simulink model "mvdr_4x4_partial_systolic"  (R2023a)
settings: Solver=FixedStepDiscrete  StartTime=0.0  StopTime=stoptime  RelTol=1e-3
InitFcn:
  | model_init
values from neighbouring files (symbols this model uses):
  diagLoading = 5e-3    (= 0.005)    [model_init.m]
  movavg_bitshift = nextpow2(windowSize)    [model_init.m]
  mvdrPipelineDelay = covMatDelay+movAvgDelay+matrixSolveDelay+normResponseDelay    [model_init.m]
  numArrayElements = 4    [model_init.m]
  reciprocalDelay = nextpow2(reciprocalin_dt.WordLength) + 1 + reciprocalin_dt.WordLength + 2      - strcmp(reciprocalin_dt.Signedness,'Signed') + 7    [model_init.m]
  sv = double(fi(signalWeights, sv_dt))    [model_init.m]
  sv_dt = fixdt(1,18,16)    [model_init.m]
  windowSize = 4096    [model_init.m]
undefined symbols (not defined in the file or in its folder): NumBits1, NumBits2
libraries: hdlsllib x17, simulink x6, dspsrcs4 x2, embsystolicmatrixops x1, embreciprocals x1
Description:
  | MVDR HDL 4x4 systolic testbench
settings Model: DataTypeOverride=Off  Creator=The MathWorks, Inc.  LastModifiedBy=tmealey
settings SolverCC: AlgebraicLoopSolver=TrustRegion
settings DataIOCC: LimitDataPoints=on  SaveFormat=Array  SaveOutput=off  SignalLogging=off  SaveTime=off
settings OptimizationCC: BlockReduction=off  ConditionallyExecuteInputs=off  DefaultParameterBehavior=Inlined  InheritOutputTypeSmallerThanSingle=on  LifeSpan=inf
settings DebuggingCC: ReadBeforeWriteMsg=DisableAll  WriteAfterWriteMsg=DisableAll  WriteAfterReadMsg=DisableAll  AlgebraicLoopMsg=error  UnderspecifiedInitializationDetection=Classic  MergeDetectMultiDrivingBlocksExec=none  SolverPrmCheckMsg=warning  SingleTaskRateTransMsg=error  ParameterPrecisionLossMsg=none  UnconnectedInputMsg=warning  UnconnectedOutputMsg=warning  UnconnectedLineMsg=warning  AllowSymbolicDim=off  SFUnexpectedBacktrackingDiag=warning  SFNoUnconditionalDefaultTransitionDiag=warning  SFExecutionAtInitializationDiag=none  ArithmeticOperatorsInVariantConditions=warning
settings HardwareCC: ProdBitPerPointer=32  ProdBitPerSizeT=32  ProdBitPerPtrDiffT=32  ProdLargestAtomicFloat=None  ProdIntDivRoundTo=Undefined  ProdEndianess=Unspecified  ProdWordSize=32  ProdHWDeviceType=ASIC/FPGA->ASIC/FPGA  TargetBitPerPointer=64  TargetBitPerSizeT=64  TargetBitPerPtrDiffT=64  TargetLongLongMode=on  TargetIntDivRoundTo=Zero  TargetEndianess=LittleEndian  TargetWordSize=64  TargetHWDeviceType=Custom Processor->MATLAB Host Computer  ProdEqTarget=off
settings ModelReferenceCC: EnableRefExpFcnMdlSchedulingChecks=on  PropagateSignalLabelsOutOfModel=off
settings SFSimCC: SimUseLocalCustomCode=off  CustomCodeUndefinedFunction=UseInterfaceOnly
settings RTWCC: RTWUseLocalCustomCode=off  DLArmComputeVersion=19.05
settings CodeAppCC: StateflowObjectComments=on
settings GRTTargetCC: TargetLangStandard=C89/C90 (ANSI)
settings ConfigComp: CovMetricSettings=dw  CovSaveCumulativeToWorkspaceVar=on  CovSaveSingleToWorkspaceVar=on  CovExternalEMLEnable=off  CovSFcnEnable=off

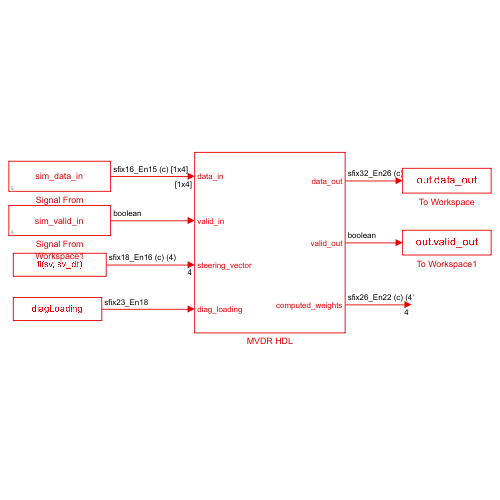
[thumbnail: Simulink's stored preview of the top-level diagram]
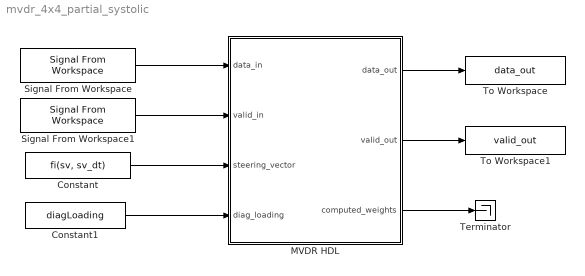
== system mvdr_4x4_partial_systolic ==
  Constant : Constant  Value=fi(sv, sv_dt)  SampleTime=1
  Constant1 : Constant  Value=diagLoading  OutDataTypeStr=matrixdivin_dt  SampleTime=-1
  MVDR HDL : Subsystem
  Signal From Workspace : dspsrcs4/Signal From Workspace  X=sim_data_in  Ts=1  nsamps=1  OutputAfterFinalValue=Setting to zero  ignoreOrWarnInputAndFrameLengths=off  OutputFrames=off
  Signal From Workspace1 : dspsrcs4/Signal From Workspace  X=sim_valid_in  Ts=1  nsamps=1  OutputAfterFinalValue=Setting to zero  ignoreOrWarnInputAndFrameLengths=off  OutputFrames=off
  Terminator : Terminator
  To Workspace : ToWorkspace  VariableName=data_out  SampleTime=-1
      settings: Save2DSignal=2-D array (concatenate along first dimension)
  To Workspace1 : ToWorkspace  VariableName=valid_out  SampleTime=-1
      settings: Save2DSignal=2-D array (concatenate along first dimension)
  wires:
  MVDR HDL/2(valid_out) -> To Workspace1/1
  MVDR HDL/1(data_out) -> To Workspace/1
  Constant/1 -> MVDR HDL/3(steering_vector)
  Signal From Workspace/1 -> MVDR HDL/1(data_in)
  Signal From Workspace1/1 -> MVDR HDL/2(valid_in)
  MVDR HDL/3(computed_weights) -> Terminator/1
  Constant1/1 -> MVDR HDL/4(diag_loading)

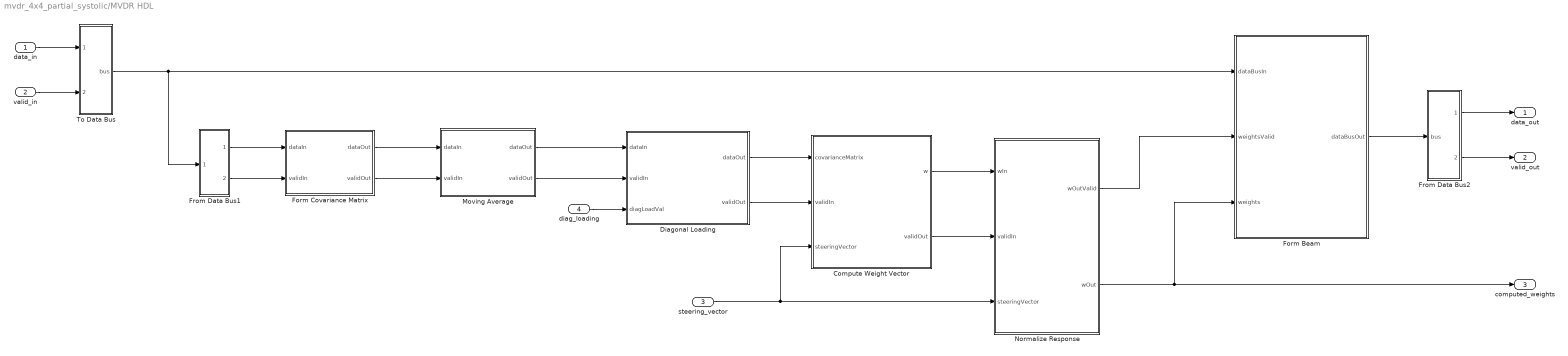
== system mvdr_4x4_partial_systolic/MVDR HDL ==
  data_in : Inport
  valid_in : Inport  Port=2
  steering_vector : Inport  Port=3
  diag_loading : Inport  Port=4
  Compute Weight Vector : Subsystem
  Diagonal Loading : Subsystem
  Form Beam : Subsystem
  Form Covariance Matrix : Subsystem
  From Data Bus1 : Subsystem
  From Data Bus2 : Subsystem
  Moving Average : Subsystem
  Normalize Response : Subsystem
  To Data Bus : Subsystem
  data_out : Outport
  valid_out : Outport  Port=2
  computed_weights : Outport  Port=3
  wires:
  valid_in/1 -> To Data Bus/2(valid)
  Form Covariance Matrix/2(validOut) -> Moving Average/2(validIn)
  Compute Weight Vector/1(w) -> Normalize Response/1(wIn)
  steering_vector/1 -> Normalize Response/3(steeringVector), Compute Weight Vector/3(steeringVector)
  data_in/1 -> To Data Bus/1(data)
  Form Covariance Matrix/1(dataOut) -> Moving Average/1(dataIn)
  To Data Bus/1(bus) -> From Data Bus1/1(bus), Form Beam/1(dataBusIn)
  Compute Weight Vector/2(validOut) -> Normalize Response/2(validIn)
  From Data Bus1/1(data) -> Form Covariance Matrix/1(dataIn)
  From Data Bus1/2(valid) -> Form Covariance Matrix/2(validIn)
  Form Beam/1(dataBusOut) -> From Data Bus2/1(bus)
  From Data Bus2/1(data) -> data_out/1
  From Data Bus2/2(valid) -> valid_out/1
  Diagonal Loading/2(validOut) -> Compute Weight Vector/2(validIn)
  Moving Average/2(validOut) -> Diagonal Loading/2(validIn)
  Moving Average/1(dataOut) -> Diagonal Loading/1(dataIn)
  Diagonal Loading/1(dataOut) -> Compute Weight Vector/1(covarianceMatrix)
  Normalize Response/2(wOut) -> computed_weights/1, Form Beam/3(weights)
  Normalize Response/1(wOutValid) -> Form Beam/2(weightsValid)
  diag_loading/1 -> Diagonal Loading/3(diagLoadVal)

== system mvdr_4x4_partial_systolic/MVDR HDL/Compute Weight Vector ==
  covarianceMatrix : Inport
  validIn : Inport  Port=2
  steeringVector : Inport  Port=3
  Complex Partial-Systolic Matrix Solve Using QR Decomposition : embsystolicmatrixops/Complex Partial-Systolic Matrix Solve Using QR Decomposition  m=4  n=4  p=1  regularizationParameter=0  OutputType=matrixdivbacksub_dt
  Constant : Constant  Value=false  SampleTime=-1
  Data Type Conversion2 : DataTypeConversion  OutDataTypeStr=matrixdivin_dt  SaturateOnIntegerOverflow=off  RndMeth=Floor
  Deserialize Output Data : Subsystem
  Reshape1 : Reshape  OutputDimensionality=Column vector (2-D)  OutputDimensions=[4,4]
  Serialize Input Data : Subsystem
  w : Outport
  validOut : Outport  Port=2
  wires:
  steeringVector/1 -> Data Type Conversion2/1
  Data Type Conversion2/1 -> Reshape1/1
  validIn/1 -> Serialize Input Data/3(validIn)
  Constant/1 -> Complex Partial-Systolic Matrix Solve Using QR Decomposition/4
  Serialize Input Data/3(validOut) -> Complex Partial-Systolic Matrix Solve Using QR Decomposition/3  "matrixSolveValidIn"
  Complex Partial-Systolic Matrix Solve Using QR Decomposition/3 -> Serialize Input Data/4(readyIn)  "matrixSolveReady"
  Serialize Input Data/1(AOut) -> Complex Partial-Systolic Matrix Solve Using QR Decomposition/1
  Reshape1/1 -> Serialize Input Data/2(BIn)
  Complex Partial-Systolic Matrix Solve Using QR Decomposition/1 -> Deserialize Output Data/1(dataIn)
  Complex Partial-Systolic Matrix Solve Using QR Decomposition/2 -> Deserialize Output Data/2(validIn)  "matrixSolveValidOut"
  Deserialize Output Data/1(dataOut) -> w/1
  Deserialize Output Data/2(validOut) -> validOut/1
  Serialize Input Data/2(BOut) -> Complex Partial-Systolic Matrix Solve Using QR Decomposition/2
  covarianceMatrix/1 -> Serialize Input Data/1(AIn)

== system mvdr_4x4_partial_systolic/MVDR HDL/Diagonal Loading ==
  dataIn : Inport
  validIn : Inport  Port=2
  diagLoadVal : Inport  Port=3
  Add : Sum
  Data Type Conversion1 : DataTypeConversion  OutDataTypeStr=matrixdivin_dt  SaturateOnIntegerOverflow=off  RndMeth=Floor
  Delay3 : Delay  DelayLength=1
  Delay6 : Delay  DelayLength=1
  Generate Loading Eye Matrix : MATLAB Function  TreatAsAtomicUnit=on
  Reshape1 : Reshape  OutputDimensions=[4,4]
  To Workspace2 : ToWorkspace  VariableName=Ecx_loaded  SampleTime=-1
      settings: Save2DSignal=2-D array (concatenate along first dimension)
  dataOut : Outport
  validOut : Outport  Port=2
  wires:
  Reshape1/1 -> To Workspace2/1
  Data Type Conversion1/1 -> dataOut/1, Reshape1/1
  Delay3/1 -> Data Type Conversion1/1
  dataIn/1 -> Add/2
  Generate Loading Eye Matrix/1(out) -> Add/1
  Add/1 -> Delay3/1
  Delay6/1 -> validOut/1
  diagLoadVal/1 -> Generate Loading Eye Matrix/1(in)
  validIn/1 -> Delay6/1

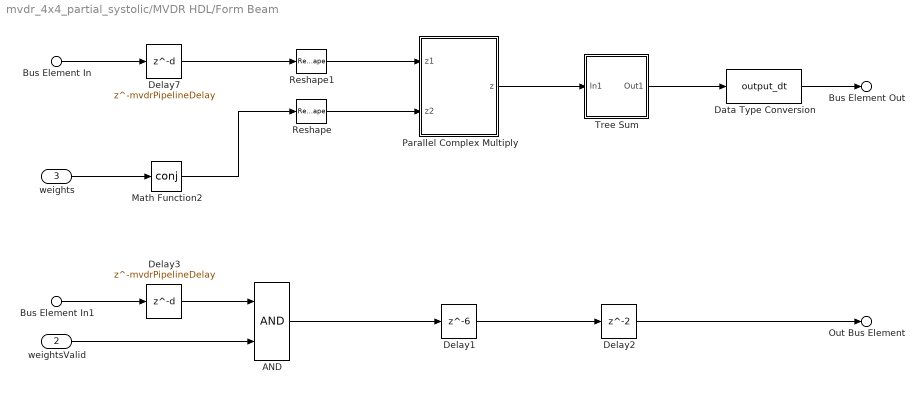
== system mvdr_4x4_partial_systolic/MVDR HDL/Form Beam ==
  Bus Element In : Inport  PortName=dataBusIn  Element=data
  Bus Element In1 : Inport  PortName=dataBusIn  Element=valid
  weightsValid : Inport  Port=2
  weights : Inport  Port=3
  AND : Logic  IconShape=distinctive  AllPortsSameDT=off  OutDataTypeStr=boolean
  Data Type Conversion : DataTypeConversion  OutDataTypeStr=output_dt  SaturateOnIntegerOverflow=off  RndMeth=Floor
  Delay1 : Delay  DelayLength=6
  Delay2 : Delay
  Delay3 : Delay  DelayLength=mvdrPipelineDelay
  Delay7 : Delay  DelayLength=mvdrPipelineDelay
  Math Function2 : Math  Operator=conj
  Parallel Complex Multiply : Subsystem  TreatAsAtomicUnit=on
  Reshape : Reshape
  Reshape1 : Reshape
  Tree Sum : Subsystem
  Bus Element Out : Outport  PortName=dataBusOut  Element=data
  Out Bus Element : Outport  PortName=dataBusOut  Element=valid
  wires:
  Parallel Complex Multiply/1(z) -> Tree Sum/1(In1)
  Tree Sum/1(Out1) -> Data Type Conversion/1
  Math Function2/1 -> Reshape/1
  weights/1 -> Math Function2/1
  Reshape/1 -> Parallel Complex Multiply/2(z2)
  Reshape1/1 -> Parallel Complex Multiply/1(z1)
  Data Type Conversion/1 -> Bus Element Out/1
  Delay2/1 -> Out Bus Element/1
  Delay1/1 -> Delay2/1
  Bus Element In1/1 -> Delay3/1
  Bus Element In/1 -> Delay7/1
  Delay7/1 -> Reshape1/1
  Delay3/1 -> AND/1
  weightsValid/1 -> AND/2
  AND/1 -> Delay1/1

== system mvdr_4x4_partial_systolic/MVDR HDL/Form Covariance Matrix ==
  dataIn : Inport
  validIn : Inport  Port=2
  Conj : Math  Operator=conj  SaturateOnIntegerOverflow=off
  Data Type Conversion : DataTypeConversion  OutDataTypeStr=covmat_dt  SaturateOnIntegerOverflow=off  RndMeth=Floor
  Data Type Conversion1 : DataTypeConversion  OutDataTypeStr=adc_dt  SaturateOnIntegerOverflow=off  RndMeth=Floor
  Delay : Delay  DelayLength=6
  Matrix Multiply Partitioned : Subsystem  TreatAsAtomicUnit=on
  Reshape : Reshape
  dataOut : Outport
  validOut : Outport  Port=2
  wires:
  validIn/1 -> Delay/1
  dataIn/1 -> Data Type Conversion1/1
  Reshape/1 -> Conj/1, Matrix Multiply Partitioned/1(x)  "x"
  Matrix Multiply Partitioned/1(C) -> Data Type Conversion/1  "x * x'"
  Delay/1 -> validOut/1
  Conj/1 -> Matrix Multiply Partitioned/2(x_conj)
  Data Type Conversion1/1 -> Reshape/1
  Data Type Conversion/1 -> dataOut/1

== system mvdr_4x4_partial_systolic/MVDR HDL/From Data Bus1 ==
  bus : Inport
  Bus Selector : BusSelector  OutputSignals=data,valid
  data : Outport
  valid : Outport  Port=2
  wires:
  bus/1 -> Bus Selector/1
  Bus Selector/1 -> data/1  "<data>"
  Bus Selector/2 -> valid/1  "<valid>"

== system mvdr_4x4_partial_systolic/MVDR HDL/From Data Bus2 ==
  bus : Inport
  Bus Selector : BusSelector  OutputSignals=data,valid
  data : Outport
  valid : Outport  Port=2
  wires:
  Bus Selector/2 -> valid/1  "<valid>"
  Bus Selector/1 -> data/1  "<data>"
  bus/1 -> Bus Selector/1

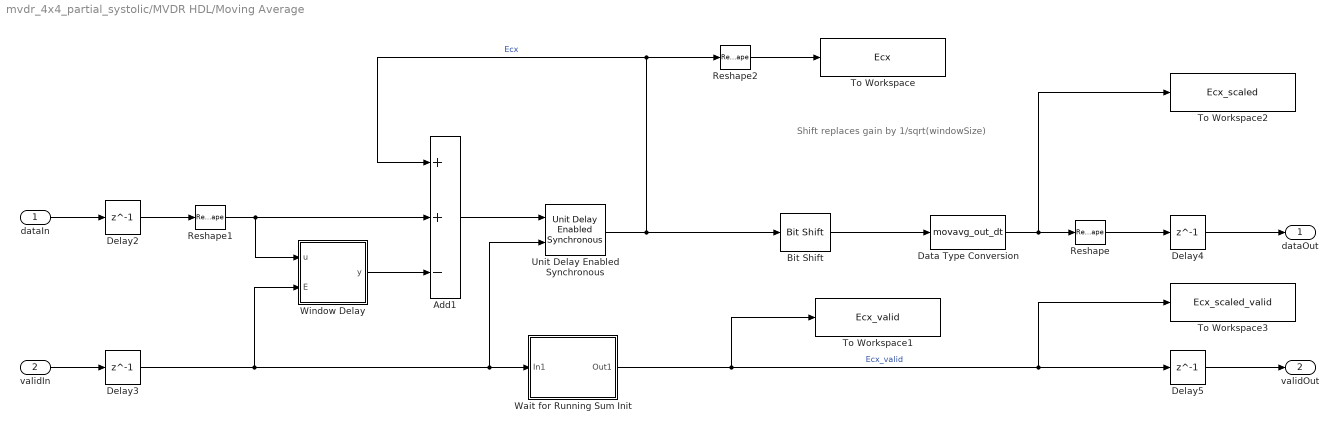
== system mvdr_4x4_partial_systolic/MVDR HDL/Moving Average ==
  note: Shift replaces gain by 1/sqrt(windowSize)
  dataIn : Inport
  validIn : Inport  Port=2
  Add1 : Sum  Inputs=++-  AccumDataTypeStr=movavg_accum_dt  OutDataTypeStr=Inherit: Same as accumulator
  Bit Shift : hdlsllib/Logic and Bit Operations/Bit Shift  mode=Shift Right Arithmetic  N=movavg_bitshift
  Data Type Conversion : DataTypeConversion  OutDataTypeStr=movavg_out_dt  SaturateOnIntegerOverflow=off  RndMeth=Floor
  Delay{2..5} (4 alike) : Delay  DelayLength=1
  Reshape : Reshape  OutputDimensionality=Customize  OutputDimensions=[4,4]
  Reshape1 : Reshape  OutputDimensions=[4,4]
  Reshape2 : Reshape  OutputDimensions=[4,4]
  To Workspace : ToWorkspace  VariableName=Ecx  SampleTime=-1
      settings: Save2DSignal=2-D array (concatenate along first dimension)
  To Workspace1 : ToWorkspace  VariableName=Ecx_valid  SampleTime=-1
      settings: Save2DSignal=2-D array (concatenate along first dimension)
  To Workspace2 : ToWorkspace  VariableName=Ecx_scaled  SampleTime=-1
      settings: Save2DSignal=2-D array (concatenate along first dimension)
  To Workspace3 : ToWorkspace  VariableName=Ecx_scaled_valid  SampleTime=-1
      settings: Save2DSignal=2-D array (concatenate along first dimension)
  Unit Delay Enabled Synchronous : hdlsllib/Discrete/Unit Delay Enabled Synchronous  InitialCondition=0.0  SampleTime=-1
  Wait for Running Sum Init : Subsystem
  Window Delay : Subsystem
  dataOut : Outport
  validOut : Outport  Port=2
  wires:
  Bit Shift/1 -> Data Type Conversion/1
  Unit Delay Enabled Synchronous/1 -> Bit Shift/1, Add1/1, Reshape2/1  "Ecx"
  Add1/1 -> Unit Delay Enabled Synchronous/1
  dataIn/1 -> Delay2/1
  validIn/1 -> Delay3/1
  Delay2/1 -> Reshape1/1
  Delay4/1 -> dataOut/1
  Delay5/1 -> validOut/1
  Delay3/1 -> Window Delay/2(E), Unit Delay Enabled Synchronous/2, Wait for Running Sum Init/1(In1)
  Wait for Running Sum Init/1(Out1) -> To Workspace1/1, To Workspace3/1, Delay5/1  "Ecx_valid"
  Data Type Conversion/1 -> To Workspace2/1, Reshape/1
  Reshape/1 -> Delay4/1
  Reshape1/1 -> Window Delay/1(u), Add1/2
  Window Delay/1(y) -> Add1/3
  Reshape2/1 -> To Workspace/1

== system mvdr_4x4_partial_systolic/MVDR HDL/Normalize Response ==
  note: This subsystem scales the weight vector to ensure unit gain in the target direction.
  wIn : Inport
  validIn : Inport  Port=2
  steeringVector : Inport  Port=3
  MVDR Weight Update : Subsystem
  Set Latch : Subsystem
  Unit Delay Enabled Synchronous : hdlsllib/Discrete/Unit Delay Enabled Synchronous  InitialCondition=0.0  SampleTime=-1
  wOutValid : Outport
  wOut : Outport  Port=2
  wires:
  steeringVector/1 -> MVDR Weight Update/1(sv)
  wIn/1 -> MVDR Weight Update/2(wp)
  MVDR Weight Update/1(w) -> Unit Delay Enabled Synchronous/1
  MVDR Weight Update/2(validOut) -> Set Latch/1(S), Unit Delay Enabled Synchronous/2
  Unit Delay Enabled Synchronous/1 -> wOut/1
  validIn/1 -> MVDR Weight Update/3(validIn)
  Set Latch/1(Q) -> wOutValid/1

== system mvdr_4x4_partial_systolic/MVDR HDL/To Data Bus ==
  data : Inport
  valid : Inport  Port=2
  Bus Creator : BusCreator  Inputs=2
  bus : Outport
  wires:
  data/1 -> Bus Creator/1  "data"
  Bus Creator/1 -> bus/1
  valid/1 -> Bus Creator/2  "valid"

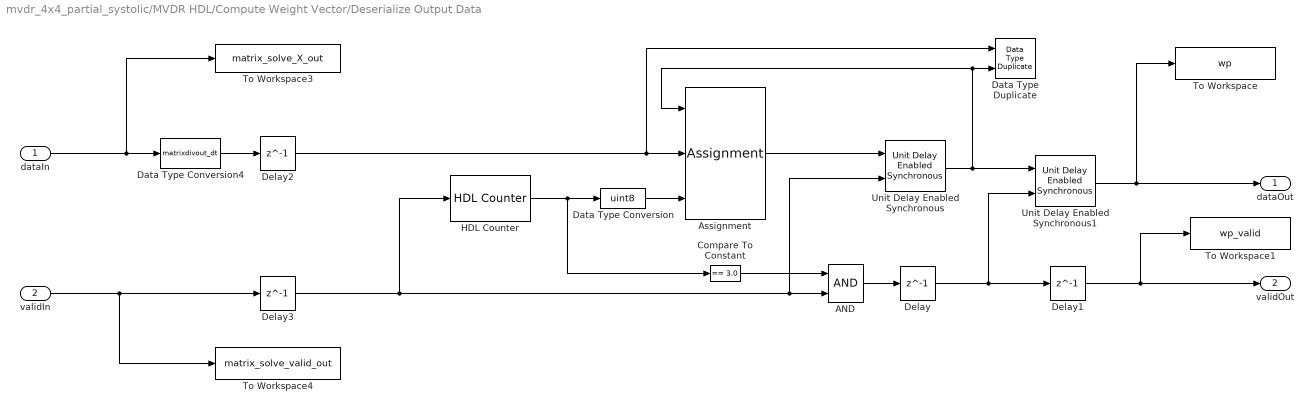
== system mvdr_4x4_partial_systolic/MVDR HDL/Compute Weight Vector/Deserialize Output Data ==
  dataIn : Inport
  validIn : Inport  Port=2
  AND : Logic  IconShape=distinctive  AllPortsSameDT=off  OutDataTypeStr=boolean
  Assignment : Assignment  IndexMode=Zero-based  DiagnosticForDimensions=Warning  IndexOptions=Index vector (port)  Indices=1  OutputSizes=4
  Compare To Constant : simulink/Logic and Bit Operations/Compare To Constant  relop===  const=3.0  OutDataTypeStr=boolean
  Data Type Duplicate : DataTypeDuplicate
  Data Type Conversion : DataTypeConversion  OutDataTypeStr=uint8  SaturateOnIntegerOverflow=off  RndMeth=Floor
  Data Type Conversion4 : DataTypeConversion  OutDataTypeStr=matrixdivout_dt  RndMeth=Convergent  SaturateOnIntegerOverflow=off
  Delay{,1..3} (4 alike) : Delay  DelayLength=1
  HDL Counter : hdlsllib/Sources/HDL Counter  CountType=Free running  CountInit=0  CountStep=1  CountMax=25  CountFromType=Initial value  CountFrom=0  CountResetPort=off  CountLoadPort=off  CountEnbPort=on  CountDirPort=off  CountHitOutputPort=off  CountDataType=Unsigned  CountWordLen=2  CountFracLen=0  CountSampTime=1
  To Workspace : ToWorkspace  VariableName=wp  SampleTime=-1
      settings: Save2DSignal=2-D array (concatenate along first dimension)
  To Workspace1 : ToWorkspace  VariableName=wp_valid  SampleTime=-1
      settings: Save2DSignal=2-D array (concatenate along first dimension)
  To Workspace3 : ToWorkspace  VariableName=matrix_solve_X_out  SampleTime=-1
      settings: Save2DSignal=2-D array (concatenate along first dimension)
  To Workspace4 : ToWorkspace  VariableName=matrix_solve_valid_out  SampleTime=-1
      settings: Save2DSignal=2-D array (concatenate along first dimension)
  Unit Delay Enabled Synchronous : hdlsllib/Discrete/Unit Delay Enabled Synchronous  InitialCondition=complex(zeros(4,1))  SampleTime=-1
  Unit Delay Enabled Synchronous1 : hdlsllib/Discrete/Unit Delay Enabled Synchronous  InitialCondition=0  SampleTime=-1
  dataOut : Outport
  validOut : Outport  Port=2
  wires:
  AND/1 -> Delay/1
  HDL Counter/1 -> Compare To Constant/1, Data Type Conversion/1
  dataIn/1 -> Data Type Conversion4/1, To Workspace3/1
  Compare To Constant/1 -> AND/1
  Delay/1 -> Delay1/1, Unit Delay Enabled Synchronous1/2
  Data Type Conversion/1 -> Assignment/3
  validIn/1 -> To Workspace4/1, Delay3/1
  Assignment/1 -> Unit Delay Enabled Synchronous/1
  Unit Delay Enabled Synchronous/1 -> Assignment/1, Data Type Duplicate/2, Unit Delay Enabled Synchronous1/1
  Delay1/1 -> To Workspace1/1, validOut/1
  Unit Delay Enabled Synchronous1/1 -> dataOut/1, To Workspace/1
  Data Type Conversion4/1 -> Delay2/1
  Delay2/1 -> Data Type Duplicate/1, Assignment/2
  Delay3/1 -> HDL Counter/1, Unit Delay Enabled Synchronous/2, AND/2

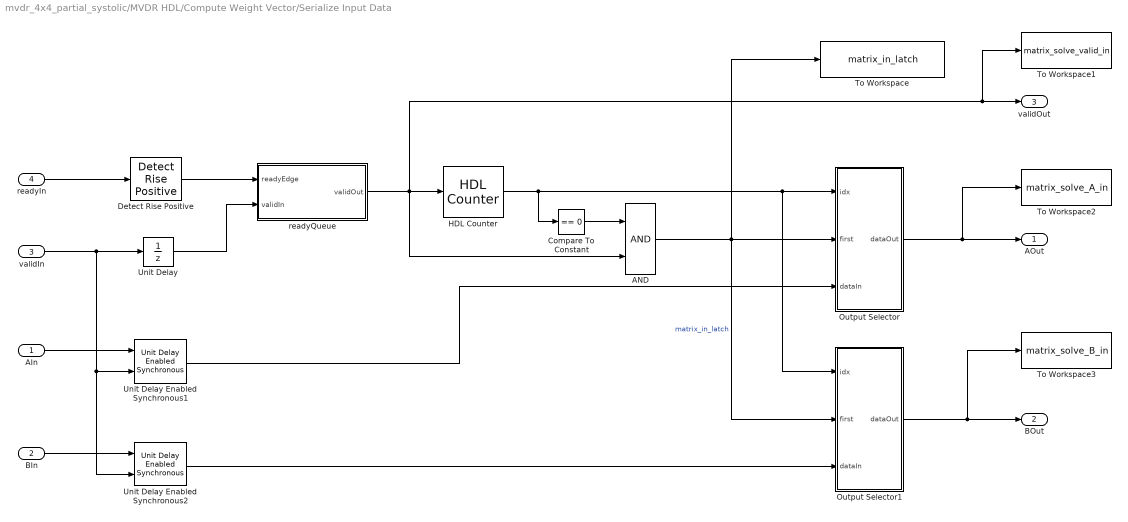
== system mvdr_4x4_partial_systolic/MVDR HDL/Compute Weight Vector/Serialize Input Data ==
  AIn : Inport
  BIn : Inport  Port=2
  validIn : Inport  Port=3
  readyIn : Inport  Port=4
  AND : Logic  IconShape=distinctive  AllPortsSameDT=off  OutDataTypeStr=boolean
  Compare To Constant : simulink/Logic and Bit Operations/Compare To Constant  relop===  const=0  OutDataTypeStr=boolean
  Detect Rise Positive : simulink/Logic and Bit Operations/Detect Rise Positive  vinit=0  OutDataTypeStr=boolean
  HDL Counter : hdlsllib/Sources/HDL Counter  CountType=Free running  CountInit=0  CountStep=1  CountMax=25  CountFromType=Initial value  CountFrom=0  CountResetPort=off  CountLoadPort=off  CountEnbPort=on  CountDirPort=off  CountHitOutputPort=off  CountDataType=Unsigned  CountWordLen=2  CountFracLen=0  CountSampTime=1
  Output Selector : Subsystem
  Output Selector1 : Subsystem
  To Workspace : ToWorkspace  VariableName=matrix_in_latch  SampleTime=-1
      settings: Save2DSignal=2-D array (concatenate along first dimension)
  To Workspace1 : ToWorkspace  VariableName=matrix_solve_valid_in  SampleTime=-1
      settings: Save2DSignal=2-D array (concatenate along first dimension)
  To Workspace2 : ToWorkspace  VariableName=matrix_solve_A_in  SampleTime=-1
      settings: Save2DSignal=2-D array (concatenate along first dimension)
  To Workspace3 : ToWorkspace  VariableName=matrix_solve_B_in  SampleTime=-1
      settings: Save2DSignal=2-D array (concatenate along first dimension)
  Unit Delay : UnitDelay  SampleTime=-1  HasFrameUpgradeWarning=on
  Unit Delay Enabled Synchronous1 : hdlsllib/Discrete/Unit Delay Enabled Synchronous  InitialCondition=0.0  SampleTime=-1
  Unit Delay Enabled Synchronous2 : hdlsllib/Discrete/Unit Delay Enabled Synchronous  InitialCondition=0.0  SampleTime=-1
  readyQueue : MATLAB Function  TreatAsAtomicUnit=on
  AOut : Outport
  BOut : Outport  Port=2
  validOut : Outport  Port=3
  wires:
  readyIn/1 -> Detect Rise Positive/1
  HDL Counter/1 -> Compare To Constant/1, Output Selector1/1(idx), Output Selector/1(idx)
  Compare To Constant/1 -> AND/1
  readyQueue/1(validOut) -> HDL Counter/1, AND/2, To Workspace1/1, validOut/1
  Detect Rise Positive/1 -> readyQueue/1(readyEdge)
  AIn/1 -> Unit Delay Enabled Synchronous1/1
  validIn/1 -> Unit Delay Enabled Synchronous2/2, Unit Delay Enabled Synchronous1/2, Unit Delay/1
  Unit Delay/1 -> readyQueue/2(validIn)
  BIn/1 -> Unit Delay Enabled Synchronous2/1
  AND/1 -> To Workspace/1, Output Selector1/2(first), Output Selector/2(first)  "matrix_in_latch"
  Unit Delay Enabled Synchronous1/1 -> Output Selector/3(dataIn)
  Output Selector/1(dataOut) -> To Workspace2/1, AOut/1
  Unit Delay Enabled Synchronous2/1 -> Output Selector1/3(dataIn)
  Output Selector1/1(dataOut) -> To Workspace3/1, BOut/1

== system mvdr_4x4_partial_systolic/MVDR HDL/Form Beam/Parallel Complex Multiply ==
  z1 : Inport  Partition=on  PartitionDimension=1  PartitionWidth=1  PartitionOffset=0
  z2 : Inport  Port=2  Partition=on  PartitionDimension=1  PartitionWidth=1  PartitionOffset=0
  For Each : ForEach  DisableCoverage=on
  HDL Complex Multiply : Subsystem  mask(HDL Complex Multiplier (3 Multiply, 5 Add)){D1=2, D2=1, D3=1, D4=1, D5=1}
      mask help:
      | Xilinx devices:
      | - Set D1 = 1 or 2 to trade off speed & FF resources
      | - Set D2-D5 = 1 to fully leverage DSP48 pipelines
      | - Use sync reset
      |
      | Intel FPGAs:
      | - Set D1 = 1 or 2 depending on device family
      | - Set D5 = 1; D2, D3, D4 = 0
      | - Use async reset
      mask init:
      | delay = D1+D2+D3+D4+D5;
      mask Display:
      | fprintf('Delay=%d',delay);
      | port_label('input',1,'z1');
      | port_label('input',2,'z2');
  z : Outport  ConcatenationDimension=1
  wires:
  z1/1 -> HDL Complex Multiply/1(In1)
  z2/1 -> HDL Complex Multiply/2(In2)
  HDL Complex Multiply/1(Out1) -> z/1

== system mvdr_4x4_partial_systolic/MVDR HDL/Form Beam/Tree Sum ==
  In1 : Inport
  Delay3 : Delay  DelayLength=ceil(log2(numArrayElements))
  Tree Sum of Elements : Sum  Inputs=+  OutDataTypeStr=Inherit: Same as first input  LockScale=on
  Out1 : Outport
  wires:
  Delay3/1 -> Out1/1
  In1/1 -> Tree Sum of Elements/1
  Tree Sum of Elements/1 -> Delay3/1

== system mvdr_4x4_partial_systolic/MVDR HDL/Form Covariance Matrix/Matrix Multiply Partitioned ==
  x : Inport
  x_conj : Inport  Port=2
  Partition x_conj : Subsystem
  Reshape : Reshape  OutputDimensionality=Customize  OutputDimensions=[4,4]
  C : Outport
  wires:
  x/1 -> Partition x_conj/1(x)
  x_conj/1 -> Partition x_conj/2(x_conj)
  Partition x_conj/1(C) -> Reshape/1
  Reshape/1 -> C/1

== system mvdr_4x4_partial_systolic/MVDR HDL/Moving Average/Wait for Running Sum Init ==
  In1 : Inport
  Compare To Constant : simulink/Logic and Bit Operations/Compare To Constant  relop=<  const=windowSize  OutDataTypeStr=boolean
  HDL Counter : hdlsllib/Sources/HDL Counter  CountType=Free running  CountInit=0  CountStep=1  CountMax=25  CountFromType=Initial value  CountFrom=0  CountResetPort=off  CountLoadPort=off  CountEnbPort=on  CountDirPort=off  CountHitOutputPort=off  CountDataType=Unsigned  CountWordLen=nextpow2(windowSize)+1  CountFracLen=0  CountSampTime=1
  Logical Operator : Logic  IconShape=distinctive  AllPortsSameDT=off  OutDataTypeStr=boolean
  Logical Operator1 : Logic  IconShape=distinctive  AllPortsSameDT=off  OutDataTypeStr=boolean
  Logical Operator2 : Logic  Operator=NOT  IconShape=distinctive  AllPortsSameDT=off  OutDataTypeStr=boolean
  Out1 : Outport
  wires:
  Logical Operator2/1 -> Logical Operator/2
  Logical Operator1/1 -> HDL Counter/1
  Compare To Constant/1 -> Logical Operator1/2, Logical Operator2/1
  Logical Operator/1 -> Out1/1
  HDL Counter/1 -> Compare To Constant/1
  In1/1 -> Logical Operator1/1, Logical Operator/1

== system mvdr_4x4_partial_systolic/MVDR HDL/Moving Average/Window Delay ==
  u : Inport
  E : Inport  Port=2
  Delay Enabled Synchronous RAM Based : Subsystem  mask{delay=windowSize-1}
      mask prompts: delay "Delay length:"
      mask init:
      | addrWidth = max(nextpow2(delay),4);
      | 
      | blk=gcb;
      | add_blk = [blk '/Add'];
      | Simulink.suppressDiagnostic(add_blk,'SimulinkFixedPoint:util:Overflowoccurred');
      mask Display:
      | blkh=gcbh;
      | delay_val = get_param(gcb,'delay');
      | try
      |     val = num2str(evalin('base',delay_val));
      | catch ME
      |     val = 'd';
      | end
      | 
      | text(0.5,0.5,['z^{-' val '}'],'texmode','on');
      | 
      | port_label('input',1,'u');
      | port_label('input',2,'E');
      | 
      | color('blue');
      | text(0.65,0.9,'RAM')
  Unit Delay Enabled Synchronous : hdlsllib/Discrete/Unit Delay Enabled Synchronous  InitialCondition=0.0  SampleTime=-1
  y : Outport
  wires:
  E/1 -> Unit Delay Enabled Synchronous/2, Delay Enabled Synchronous RAM Based/2(E)
  u/1 -> Delay Enabled Synchronous RAM Based/1(u)
  Delay Enabled Synchronous RAM Based/1(y) -> Unit Delay Enabled Synchronous/1
  Unit Delay Enabled Synchronous/1 -> y/1

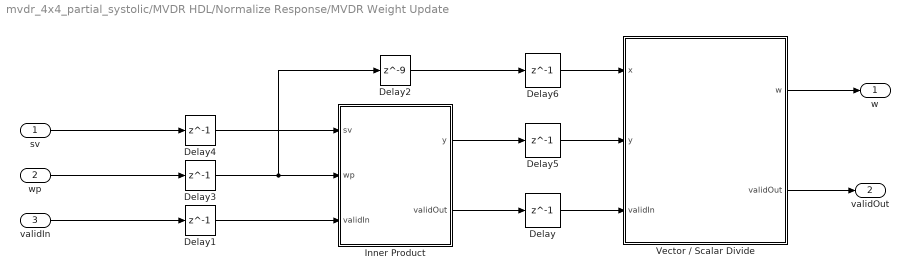
== system mvdr_4x4_partial_systolic/MVDR HDL/Normalize Response/MVDR Weight Update ==
  sv : Inport
  wp : Inport  Port=2
  validIn : Inport  Port=3
  Delay{,1,3..6} (6 alike) : Delay  DelayLength=1
  Delay2 : Delay  DelayLength=9
  Inner Product : Subsystem
  Vector / Scalar Divide : Subsystem
  w : Outport
  validOut : Outport  Port=2
  wires:
  wp/1 -> Delay3/1
  Vector / Scalar Divide/1(w) -> w/1
  Delay4/1 -> Inner Product/1(sv)
  Inner Product/1(y) -> Delay5/1
  Delay6/1 -> Vector / Scalar Divide/1(x)
  Delay/1 -> Vector / Scalar Divide/3(validIn)
  sv/1 -> Delay4/1
  Delay3/1 -> Delay2/1, Inner Product/2(wp)
  Delay5/1 -> Vector / Scalar Divide/2(y)
  Inner Product/2(validOut) -> Delay/1
  validIn/1 -> Delay1/1
  Vector / Scalar Divide/2(validOut) -> validOut/1
  Delay1/1 -> Inner Product/3(validIn)
  Delay2/1 -> Delay6/1

== system mvdr_4x4_partial_systolic/MVDR HDL/Normalize Response/Set Latch ==
  S : Inport
  Logical Operator5 : Logic  Operator=OR  IconShape=distinctive  AllPortsSameDT=off  OutDataTypeStr=boolean
  Unit Delay : UnitDelay  SampleTime=-1  HasFrameUpgradeWarning=on
  Q : Outport  VectorParamsAs1DForOutWhenUnconnected=off
  wires:
  S/1 -> Logical Operator5/1
  Logical Operator5/1 -> Unit Delay/1
  Unit Delay/1 -> Logical Operator5/2, Q/1

== system mvdr_4x4_partial_systolic/MVDR HDL/Compute Weight Vector/Serialize Input Data/Output Selector ==
  idx : Inport
  first : Inport  Port=2
  dataIn : Inport  Port=3
  Multiport Switch : MultiPortSwitch  DataPortOrder=Zero-based contiguous  Inputs=4  zeroidx=on  SaturateOnIntegerOverflow=off  InputSameDT=off
  Row 1 : Selector  NumberOfDimensions=2  InputPortWidth=3  IndexOptions=Index vector (dialog),Select all  Indices=1,1  OutputSizes=1,1
  Row 2 : Selector  NumberOfDimensions=2  InputPortWidth=3  IndexOptions=Index vector (dialog),Select all  Indices=2,1  OutputSizes=1,1
  Row 3 : Selector  NumberOfDimensions=2  InputPortWidth=3  IndexOptions=Index vector (dialog),Select all  Indices=3,1  OutputSizes=1,1
  Row 4 : Selector  NumberOfDimensions=2  InputPortWidth=3  IndexOptions=Index vector (dialog),Select all  Indices=4,1  OutputSizes=1,1
  Unit Delay Enabled Synchronous : hdlsllib/Discrete/Unit Delay Enabled Synchronous  InitialCondition=0.0  SampleTime=-1
  dataOut : Outport
  wires:
  Row 1/1 -> Multiport Switch/2
  Row 4/1 -> Multiport Switch/5
  Unit Delay Enabled Synchronous/1 -> Row 4/1, Row 3/1, Row 2/1
  dataIn/1 -> Unit Delay Enabled Synchronous/1, Row 1/1
  Row 2/1 -> Multiport Switch/3
  idx/1 -> Multiport Switch/1
  Row 3/1 -> Multiport Switch/4
  Multiport Switch/1 -> dataOut/1
  first/1 -> Unit Delay Enabled Synchronous/2

== system mvdr_4x4_partial_systolic/MVDR HDL/Compute Weight Vector/Serialize Input Data/Output Selector1 ==
  idx : Inport
  first : Inport  Port=2
  dataIn : Inport  Port=3
  Multiport Switch : MultiPortSwitch  DataPortOrder=Zero-based contiguous  Inputs=4  zeroidx=on  SaturateOnIntegerOverflow=off  InputSameDT=off
  Row 1 : Selector  NumberOfDimensions=2  InputPortWidth=3  IndexOptions=Index vector (dialog),Select all  Indices=1,1  OutputSizes=1,1
  Row 2 : Selector  NumberOfDimensions=2  InputPortWidth=3  IndexOptions=Index vector (dialog),Select all  Indices=2,1  OutputSizes=1,1
  Row 3 : Selector  NumberOfDimensions=2  InputPortWidth=3  IndexOptions=Index vector (dialog),Select all  Indices=3,1  OutputSizes=1,1
  Row 4 : Selector  NumberOfDimensions=2  InputPortWidth=3  IndexOptions=Index vector (dialog),Select all  Indices=4,1  OutputSizes=1,1
  Unit Delay Enabled Synchronous : hdlsllib/Discrete/Unit Delay Enabled Synchronous  InitialCondition=0.0  SampleTime=-1
  dataOut : Outport
  wires:
  first/1 -> Unit Delay Enabled Synchronous/2
  Multiport Switch/1 -> dataOut/1
  Row 3/1 -> Multiport Switch/4
  idx/1 -> Multiport Switch/1
  Row 2/1 -> Multiport Switch/3
  dataIn/1 -> Row 1/1, Unit Delay Enabled Synchronous/1
  Unit Delay Enabled Synchronous/1 -> Row 2/1, Row 3/1, Row 4/1
  Row 4/1 -> Multiport Switch/5
  Row 1/1 -> Multiport Switch/2

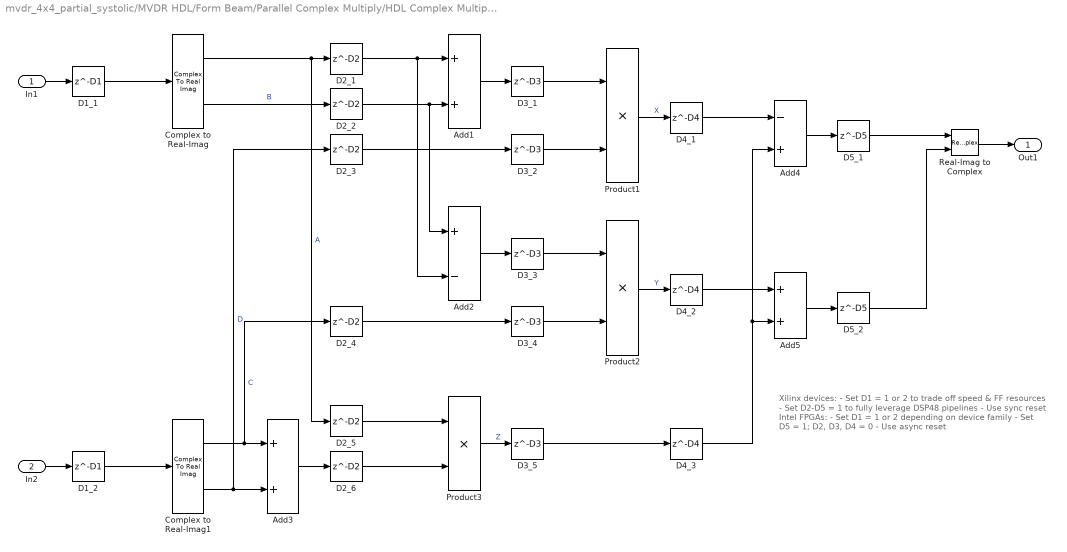
== system mvdr_4x4_partial_systolic/MVDR HDL/Form Beam/Parallel Complex Multiply/HDL Complex Multiply ==
  note: Xilinx devices:
      | - Set D1 = 1 or 2 to trade off speed & FF resources
      | - Set D2-D5 = 1 to fully leverage DSP48 pipelines
      | - Use sync reset
      |
      | Intel FPGAs:
      | - Set D1 = 1 or 2 depending on device family
      | - Set D5 = 1; D2, D3, D4 = 0
      | - Use async reset
  In1 : Inport
  In2 : Inport  Port=2
  Add1 : Sum
  Add2 : Sum  Inputs=+-
  Add3 : Sum
  Add4 : Sum  Inputs=-+
  Add5 : Sum
  Complex to Real-Imag : ComplexToRealImag
  Complex to Real-Imag1 : ComplexToRealImag
  D1_1 : Delay  DelayLength=D1
  D1_2 : Delay  DelayLength=D1
  D2_{1..6} (6 alike) : Delay  DelayLength=D2
  D3_{1..5} (5 alike) : Delay  DelayLength=D3
  D4_1 : Delay  DelayLength=D4
  D4_2 : Delay  DelayLength=D4
  D4_3 : Delay  DelayLength=D4
  D5_1 : Delay  DelayLength=D5
  D5_2 : Delay  DelayLength=D5
  Product1 : Product
  Product2 : Product
  Product3 : Product
  Real-Imag to Complex : RealImagToComplex
  Out1 : Outport  VectorParamsAs1DForOutWhenUnconnected=off
  wires:
  Real-Imag to Complex/1 -> Out1/1
  In2/1 -> D1_2/1
  Complex to Real-Imag1/1 -> Add3/1, D2_4/1  "C"
  Complex to Real-Imag1/2 -> Add3/2, D2_3/1  "D"
  Product1/1 -> D4_1/1  "X"
  Product2/1 -> D4_2/1  "Y"
  Product3/1 -> D3_5/1  "Z"
  Add4/1 -> D5_1/1
  Add5/1 -> D5_2/1
  D5_1/1 -> Real-Imag to Complex/1
  D5_2/1 -> Real-Imag to Complex/2
  D4_1/1 -> Add4/1
  D4_2/1 -> Add5/1
  D3_5/1 -> D4_3/1
  Add1/1 -> D3_1/1
  Add3/1 -> D2_6/1
  Add2/1 -> D3_3/1
  Complex to Real-Imag/1 -> D2_5/1, D2_1/1  "A"
  Complex to Real-Imag/2 -> D2_2/1  "B"
  D3_1/1 -> Product1/1
  D2_6/1 -> Product3/2
  D3_3/1 -> Product2/1
  D4_3/1 -> Add4/2, Add5/2
  D3_4/1 -> Product2/2
  D3_2/1 -> Product1/2
  D2_4/1 -> D3_4/1
  D2_3/1 -> D3_2/1
  D2_5/1 -> Product3/1
  D2_2/1 -> Add1/2, Add2/1
  D2_1/1 -> Add2/2, Add1/1
  In1/1 -> D1_1/1
  D1_1/1 -> Complex to Real-Imag/1
  D1_2/1 -> Complex to Real-Imag1/1

== system mvdr_4x4_partial_systolic/MVDR HDL/Form Covariance Matrix/Matrix Multiply Partitioned/Partition x_conj ==
  x : Inport
  x_conj : Inport  Port=2  Partition=on  PartitionDimension=1  PartitionWidth=1  PartitionOffset=0
  For Each : ForEach  DisableCoverage=on
  Partition x : Subsystem  TreatAsAtomicUnit=on
  C : Outport  ConcatenationDimension=1
  wires:
  x_conj/1 -> Partition x/2(x_conj_elem)
  x/1 -> Partition x/1(x)
  Partition x/1(C_col) -> C/1

== system mvdr_4x4_partial_systolic/MVDR HDL/Moving Average/Window Delay/Delay Enabled Synchronous RAM Based ==
  u : Inport
  E : Inport  Port=2
  Add : Sum  Inputs=++-  OutDataTypeStr=Inherit: Same as accumulator
  Constant1 : Constant  OutDataTypeStr=Inherit: Inherit via back propagation  SampleTime=-1
  Constant2 : Constant  Value=delay  OutDataTypeStr=Inherit: Inherit via back propagation  SampleTime=-1
  HDL Counter : hdlsllib/Sources/HDL Counter  CountType=Free running  CountInit=0  CountStep=1  CountMax=25  CountFromType=Initial value  CountFrom=0  CountResetPort=off  CountLoadPort=off  CountEnbPort=on  CountDirPort=off  CountHitOutputPort=off  CountDataType=Unsigned  CountWordLen=addrWidth  CountFracLen=0  CountSampTime=-1
  Simple Dual Port RAM System : hdlsllib/HDL RAMs/Simple Dual Port RAM System  RAMType=Simple dual port  WriteOutputValue=New data  RAMInitialValue=0  SimulateUsing=Code generation
  Switch1 : Switch  Criteria=u2 ~= 0  SaturateOnIntegerOverflow=off  InputSameDT=off
  Zero on Initial Delay : Subsystem
  out_prev : hdlsllib/Discrete/Unit Delay Enabled Synchronous  InitialCondition=0.0  SampleTime=-1
  read_prev : Delay  DelayLength=1
  y : Outport
  wires:
  read_prev/1 -> Switch1/2, out_prev/2
  Zero on Initial Delay/1(dout) -> Switch1/1, out_prev/1
  Simple Dual Port RAM System/1 -> Zero on Initial Delay/1(ram_dout)
  E/1 -> HDL Counter/1, Zero on Initial Delay/2(en), read_prev/1, Simple Dual Port RAM System/3
  out_prev/1 -> Switch1/3
  Switch1/1 -> y/1
  Constant2/1 -> Add/3
  Constant1/1 -> Add/2
  u/1 -> Simple Dual Port RAM System/1
  Add/1 -> Simple Dual Port RAM System/4
  HDL Counter/1 -> Add/1, Simple Dual Port RAM System/2

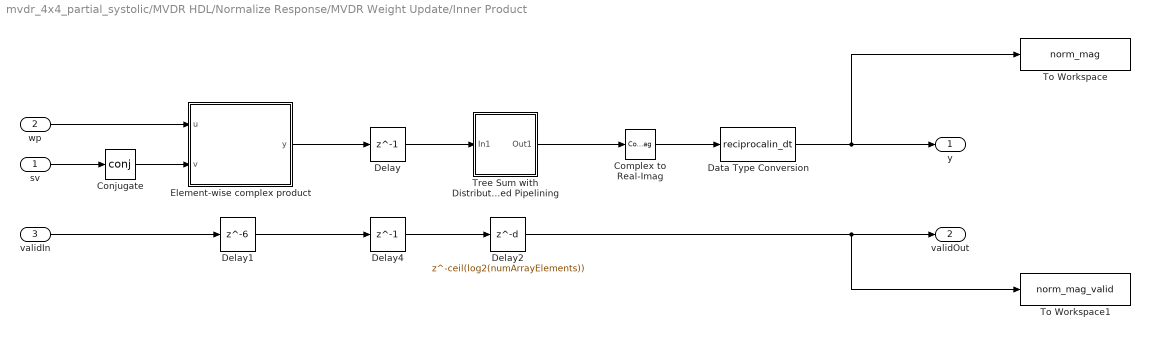
== system mvdr_4x4_partial_systolic/MVDR HDL/Normalize Response/MVDR Weight Update/Inner Product ==
  sv : Inport
  wp : Inport  Port=2
  validIn : Inport  Port=3
  Complex to Real-Imag : ComplexToRealImag  Output=Real
  Conjugate : Math  Operator=conj  SignedPower=on  RndMeth=Zero
  Data Type Conversion : DataTypeConversion  OutDataTypeStr=reciprocalin_dt  SaturateOnIntegerOverflow=off  RndMeth=Floor
  Delay : Delay  DelayLength=1
  Delay1 : Delay  DelayLength=6
  Delay2 : Delay  DelayLength=ceil(log2(numArrayElements))
  Delay4 : Delay  DelayLength=1
  Element-wise complex product : Subsystem  TreatAsAtomicUnit=on
  To Workspace : ToWorkspace  VariableName=norm_mag  SampleTime=-1
      settings: Save2DSignal=2-D array (concatenate along first dimension)
  To Workspace1 : ToWorkspace  VariableName=norm_mag_valid  SampleTime=-1
      settings: Save2DSignal=2-D array (concatenate along first dimension)
  Tree Sum with Distributed Pipelining : Subsystem
  y : Outport
  validOut : Outport  Port=2
  wires:
  sv/1 -> Conjugate/1
  validIn/1 -> Delay1/1
  Delay1/1 -> Delay4/1
  Delay4/1 -> Delay2/1
  wp/1 -> Element-wise complex product/1(u)
  Delay/1 -> Tree Sum with Distributed Pipelining/1(In1)
  Complex to Real-Imag/1 -> Data Type Conversion/1
  Element-wise complex product/1(y) -> Delay/1
  Delay2/1 -> validOut/1, To Workspace1/1
  Tree Sum with Distributed Pipelining/1(Out1) -> Complex to Real-Imag/1
  Data Type Conversion/1 -> y/1, To Workspace/1
  Conjugate/1 -> Element-wise complex product/2(v)

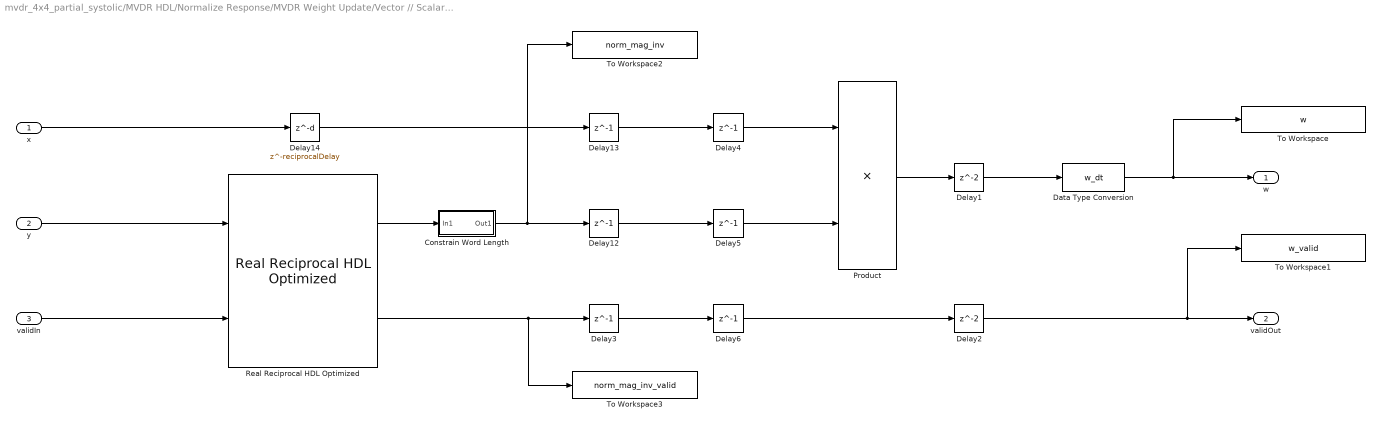
== system mvdr_4x4_partial_systolic/MVDR HDL/Normalize Response/MVDR Weight Update/Vector // Scalar Divide ==
  x : Inport
  y : Inport  Port=2
  validIn : Inport  Port=3
  Constrain Word Length : Subsystem  mask(Constrain Word Length){WL=18}
      mask prompts: WL "Maximum word length:"
      mask help: Output word length will not exceed the specified value.
      mask Display: fprintf('WL <= %d',WL);
  Data Type Conversion : DataTypeConversion  OutDataTypeStr=w_dt  SaturateOnIntegerOverflow=off  RndMeth=Floor
  Delay1 : Delay
  Delay{3..6,12..13} (6 alike) : Delay  DelayLength=1
  Delay14 : Delay  DelayLength=reciprocalDelay
  Delay2 : Delay
  Product : Product
  Real Reciprocal HDL Optimized : embreciprocals/Real Reciprocal HDL Optimized  OutputType=reciprocalout_dt
      settings: LibrarySourceBlock=embeddedMatrixLib/Math Operations/Real Reciprocal HDL Optimized
  To Workspace : ToWorkspace  VariableName=w  SampleTime=-1
      settings: Save2DSignal=2-D array (concatenate along first dimension)
  To Workspace1 : ToWorkspace  VariableName=w_valid  SampleTime=-1
      settings: Save2DSignal=2-D array (concatenate along first dimension)
  To Workspace2 : ToWorkspace  VariableName=norm_mag_inv  SampleTime=-1
      settings: Save2DSignal=2-D array (concatenate along first dimension)
  To Workspace3 : ToWorkspace  VariableName=norm_mag_inv_valid  SampleTime=-1
      settings: Save2DSignal=2-D array (concatenate along first dimension)
  w : Outport
  validOut : Outport  Port=2
  wires:
  y/1 -> Real Reciprocal HDL Optimized/1
  Real Reciprocal HDL Optimized/1 -> Constrain Word Length/1(In1)
  validIn/1 -> Real Reciprocal HDL Optimized/2
  Product/1 -> Delay1/1
  x/1 -> Delay14/1
  Delay14/1 -> Delay13/1
  Constrain Word Length/1(Out1) -> To Workspace2/1, Delay12/1
  Real Reciprocal HDL Optimized/2 -> To Workspace3/1, Delay3/1
  Delay2/1 -> To Workspace1/1, validOut/1
  Delay1/1 -> Data Type Conversion/1
  Data Type Conversion/1 -> To Workspace/1, w/1
  Delay4/1 -> Product/1
  Delay13/1 -> Delay4/1
  Delay5/1 -> Product/2
  Delay12/1 -> Delay5/1
  Delay3/1 -> Delay6/1
  Delay6/1 -> Delay2/1

== system mvdr_4x4_partial_systolic/MVDR HDL/Form Covariance Matrix/Matrix Multiply Partitioned/Partition x_conj/Partition x ==
  x : Inport  Partition=on  PartitionDimension=1  PartitionWidth=1  PartitionOffset=0
  x_conj_elem : Inport  Port=2
  For Each : ForEach  DisableCoverage=on
  HDL Complex Multiply : Subsystem  mask(HDL Complex Multiplier (3 Multiply, 5 Add)){D1=2, D2=1, D3=1, D4=1, D5=1}
      mask help:
      | Xilinx devices:
      | - Set D1 = 1 or 2 to trade off speed & FF resources
      | - Set D2-D5 = 1 to fully leverage DSP48 pipelines
      | - Use sync reset
      |
      | Intel FPGAs:
      | - Set D1 = 1 or 2 depending on device family
      | - Set D5 = 1; D2, D3, D4 = 0
      | - Use async reset
      mask init:
      | delay = D1+D2+D3+D4+D5;
      mask Display:
      | fprintf('Delay=%d',delay);
      | port_label('input',1,'z1');
      | port_label('input',2,'z2');
  C_col : Outport  ConcatenationDimension=1
  wires:
  x/1 -> HDL Complex Multiply/1(In1)
  x_conj_elem/1 -> HDL Complex Multiply/2(In2)
  HDL Complex Multiply/1(Out1) -> C_col/1

== system mvdr_4x4_partial_systolic/MVDR HDL/Moving Average/Window Delay/Delay Enabled Synchronous RAM Based/Zero on Initial Delay ==
  ram_dout : Inport
  en : Inport  Port=2
  AND : Logic  IconShape=distinctive  AllPortsSameDT=off  OutDataTypeStr=boolean
  Compare To Constant : simulink/Logic and Bit Operations/Compare To Constant  relop===  const=delay  OutDataTypeStr=boolean
  HDL Counter1 : hdlsllib/Sources/HDL Counter  CountType=Free running  CountInit=0  CountStep=1  CountMax=25  CountFromType=Initial value  CountFrom=0  CountResetPort=off  CountLoadPort=off  CountEnbPort=on  CountDirPort=off  CountHitOutputPort=off  CountDataType=Unsigned  CountWordLen=addrWidth  CountFracLen=0  CountSampTime=-1
  NOT : Logic  Operator=NOT  IconShape=distinctive  AllPortsSameDT=off  OutDataTypeStr=boolean
  Switch : Switch  Criteria=u2 ~= 0  SaturateOnIntegerOverflow=off  InputSameDT=off
  Zeros Like : MATLAB Function  TreatAsAtomicUnit=on  mask(Zeros Like){matchInputSize=on, outputSizeUser=[1 1]}
      mask prompts: matchInputSize "Match input size?"; outputSizeUser "Output size:"
      mask help: Creates a constant 0 signal with the same datatype as the input. Optionally match the size of the input or specify the output size.
      mask init:
      | if isscalar(outputSizeUser)
      |     outputSize = [outputSizeUser 1];
      | else
      |     outputSize = outputSizeUser;
      | end
  dout : Outport
  wires:
  en/1 -> AND/1
  ram_dout/1 -> Switch/1, Zeros Like/1(u)
  AND/1 -> HDL Counter1/1
  Zeros Like/1(y) -> Switch/3
  NOT/1 -> AND/2
  Compare To Constant/1 -> NOT/1, Switch/2
  HDL Counter1/1 -> Compare To Constant/1
  Switch/1 -> dout/1

== system mvdr_4x4_partial_systolic/MVDR HDL/Normalize Response/MVDR Weight Update/Inner Product/Element-wise complex product ==
  u : Inport  Partition=on  PartitionDimension=1  PartitionWidth=1  PartitionOffset=0
  v : Inport  Port=2  Partition=on  PartitionDimension=1  PartitionWidth=1  PartitionOffset=0
  For Each : ForEach  DisableCoverage=on
  HDL Complex Multiply : Subsystem  mask(HDL Complex Multiplier (3 Multiply, 5 Add)){D1=2, D2=1, D3=1, D4=1, D5=1}
      mask help:
      | Xilinx devices:
      | - Set D1 = 1 or 2 to trade off speed & FF resources
      | - Set D2-D5 = 1 to fully leverage DSP48 pipelines
      | - Use sync reset
      |
      | Intel FPGAs:
      | - Set D1 = 1 or 2 depending on device family
      | - Set D5 = 1; D2, D3, D4 = 0
      | - Use async reset
      mask init:
      | delay = D1+D2+D3+D4+D5;
      mask Display:
      | fprintf('Pipelined\nComplex Multiply\nLatency=%d',delay);
      | port_label('input',1,'z1');
      | port_label('input',2,'z2');
  y : Outport  ConcatenationDimension=1
  wires:
  v/1 -> HDL Complex Multiply/2(In2)
  u/1 -> HDL Complex Multiply/1(In1)
  HDL Complex Multiply/1(Out1) -> y/1

== system mvdr_4x4_partial_systolic/MVDR HDL/Normalize Response/MVDR Weight Update/Inner Product/Tree Sum with Distributed Pipelining ==
  In1 : Inport
  Delay3 : Delay  DelayLength=ceil(log2(numArrayElements))
  Tree Sum of Elements : Sum  Inputs=+  OutDataTypeStr=Inherit: Same as first input  LockScale=on
  Out1 : Outport
  wires:
  Delay3/1 -> Out1/1
  In1/1 -> Tree Sum of Elements/1
  Tree Sum of Elements/1 -> Delay3/1

== system mvdr_4x4_partial_systolic/MVDR HDL/Normalize Response/MVDR Weight Update/Vector // Scalar Divide/Constrain Word Length ==
  In1 : Inport
  Constant : Constant  Value=0  OutDataTypeStr=fixdt(0,WL,0)  SampleTime=-1
  Data Type Propagation : simulink/Signal Attributes/Data Type Propagation  PropDataType=fixdt(1, 16)  IfRefDouble=double  IfRefSingle=single  IsSigned=IsSigned1  NumBitsBase=min([NumBits1 NumBits2])  NumBitsMult=1  NumBitsAdd=0  NumBitsAllowFinal=1:128  PropScaling=2^-10  ValuesUsedBestPrec=[5 -7]  SlopeBase=PosRange1  SlopeMult=1  SlopeAdd=0  BiasBase=Bias1  BiasMult=1  BiasAdd=0
  Data Type Conversion : DataTypeConversion  SaturateOnIntegerOverflow=off  RndMeth=Floor
  Out1 : Outport
  wires:
  Constant/1 -> Data Type Propagation/2
  Data Type Conversion/1 -> Out1/1, Data Type Propagation/3
  In1/1 -> Data Type Conversion/1, Data Type Propagation/1

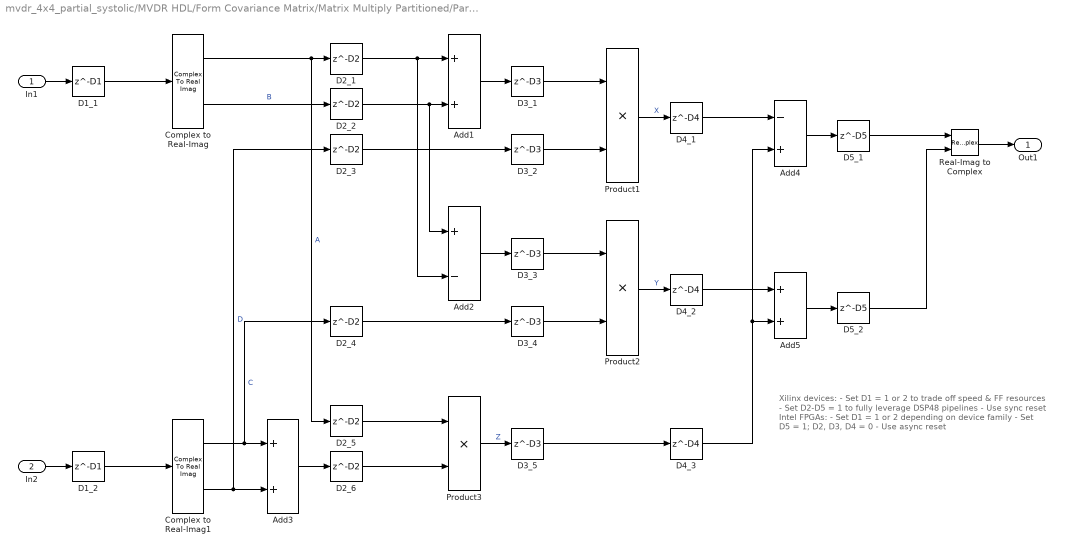
== system mvdr_4x4_partial_systolic/MVDR HDL/Form Covariance Matrix/Matrix Multiply Partitioned/Partition x_conj/Partition x/HDL Complex Multiply ==
  note: Xilinx devices:
      | - Set D1 = 1 or 2 to trade off speed & FF resources
      | - Set D2-D5 = 1 to fully leverage DSP48 pipelines
      | - Use sync reset
      |
      | Intel FPGAs:
      | - Set D1 = 1 or 2 depending on device family
      | - Set D5 = 1; D2, D3, D4 = 0
      | - Use async reset
  In1 : Inport
  In2 : Inport  Port=2
  Add1 : Sum
  Add2 : Sum  Inputs=+-
  Add3 : Sum
  Add4 : Sum  Inputs=-+
  Add5 : Sum
  Complex to Real-Imag : ComplexToRealImag
  Complex to Real-Imag1 : ComplexToRealImag
  D1_1 : Delay  DelayLength=D1
  D1_2 : Delay  DelayLength=D1
  D2_{1..6} (6 alike) : Delay  DelayLength=D2
  D3_{1..5} (5 alike) : Delay  DelayLength=D3
  D4_1 : Delay  DelayLength=D4
  D4_2 : Delay  DelayLength=D4
  D4_3 : Delay  DelayLength=D4
  D5_1 : Delay  DelayLength=D5
  D5_2 : Delay  DelayLength=D5
  Product1 : Product
  Product2 : Product
  Product3 : Product
  Real-Imag to Complex : RealImagToComplex
  Out1 : Outport  VectorParamsAs1DForOutWhenUnconnected=off
  wires:
  Real-Imag to Complex/1 -> Out1/1
  In2/1 -> D1_2/1
  Complex to Real-Imag1/1 -> Add3/1, D2_4/1  "C"
  Complex to Real-Imag1/2 -> Add3/2, D2_3/1  "D"
  Product1/1 -> D4_1/1  "X"
  Product2/1 -> D4_2/1  "Y"
  Product3/1 -> D3_5/1  "Z"
  Add4/1 -> D5_1/1
  Add5/1 -> D5_2/1
  D5_1/1 -> Real-Imag to Complex/1
  D5_2/1 -> Real-Imag to Complex/2
  D4_1/1 -> Add4/1
  D4_2/1 -> Add5/1
  D3_5/1 -> D4_3/1
  Add1/1 -> D3_1/1
  Add3/1 -> D2_6/1
  Add2/1 -> D3_3/1
  Complex to Real-Imag/1 -> D2_5/1, D2_1/1  "A"
  Complex to Real-Imag/2 -> D2_2/1  "B"
  D3_1/1 -> Product1/1
  D2_6/1 -> Product3/2
  D3_3/1 -> Product2/1
  D4_3/1 -> Add4/2, Add5/2
  D3_4/1 -> Product2/2
  D3_2/1 -> Product1/2
  D2_4/1 -> D3_4/1
  D2_3/1 -> D3_2/1
  D2_5/1 -> Product3/1
  D2_2/1 -> Add1/2, Add2/1
  D2_1/1 -> Add2/2, Add1/1
  In1/1 -> D1_1/1
  D1_1/1 -> Complex to Real-Imag/1
  D1_2/1 -> Complex to Real-Imag1/1

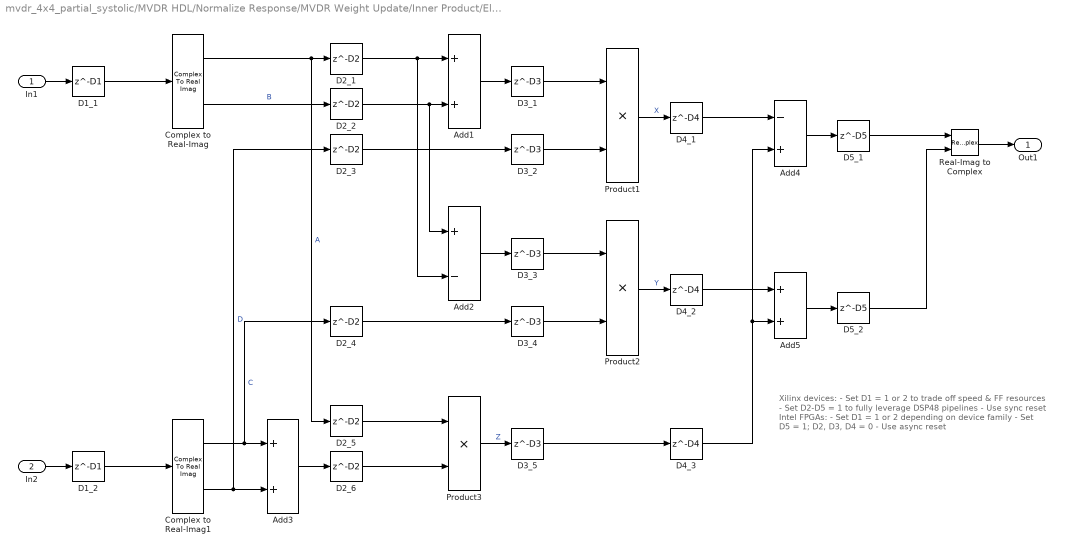
== system mvdr_4x4_partial_systolic/MVDR HDL/Normalize Response/MVDR Weight Update/Inner Product/Element-wise complex product/HDL Complex Multiply ==
  note: Xilinx devices:
      | - Set D1 = 1 or 2 to trade off speed & FF resources
      | - Set D2-D5 = 1 to fully leverage DSP48 pipelines
      | - Use sync reset
      |
      | Intel FPGAs:
      | - Set D1 = 1 or 2 depending on device family
      | - Set D5 = 1; D2, D3, D4 = 0
      | - Use async reset
  In1 : Inport
  In2 : Inport  Port=2
  Add1 : Sum
  Add2 : Sum  Inputs=+-
  Add3 : Sum
  Add4 : Sum  Inputs=-+
  Add5 : Sum
  Complex to Real-Imag : ComplexToRealImag
  Complex to Real-Imag1 : ComplexToRealImag
  D1_1 : Delay  DelayLength=D1
  D1_2 : Delay  DelayLength=D1
  D2_{1..6} (6 alike) : Delay  DelayLength=D2
  D3_{1..5} (5 alike) : Delay  DelayLength=D3
  D4_1 : Delay  DelayLength=D4
  D4_2 : Delay  DelayLength=D4
  D4_3 : Delay  DelayLength=D4
  D5_1 : Delay  DelayLength=D5
  D5_2 : Delay  DelayLength=D5
  Product1 : Product
  Product2 : Product
  Product3 : Product
  Real-Imag to Complex : RealImagToComplex
  Out1 : Outport  VectorParamsAs1DForOutWhenUnconnected=off
  wires:
  D1_2/1 -> Complex to Real-Imag1/1
  D1_1/1 -> Complex to Real-Imag/1
  In1/1 -> D1_1/1
  D2_1/1 -> Add1/1, Add2/2
  D2_2/1 -> Add2/1, Add1/2
  D2_5/1 -> Product3/1
  D2_3/1 -> D3_2/1
  D2_4/1 -> D3_4/1
  D3_2/1 -> Product1/2
  D3_4/1 -> Product2/2
  D4_3/1 -> Add5/2, Add4/2
  D3_3/1 -> Product2/1
  D2_6/1 -> Product3/2
  D3_1/1 -> Product1/1
  Complex to Real-Imag/2 -> D2_2/1  "B"
  Complex to Real-Imag/1 -> D2_1/1, D2_5/1  "A"
  Add2/1 -> D3_3/1
  Add3/1 -> D2_6/1
  Add1/1 -> D3_1/1
  D3_5/1 -> D4_3/1
  D4_2/1 -> Add5/1
  D4_1/1 -> Add4/1
  D5_2/1 -> Real-Imag to Complex/2
  D5_1/1 -> Real-Imag to Complex/1
  Add5/1 -> D5_2/1
  Add4/1 -> D5_1/1
  Product3/1 -> D3_5/1  "Z"
  Product2/1 -> D4_2/1  "Y"
  Product1/1 -> D4_1/1  "X"
  Complex to Real-Imag1/2 -> D2_3/1, Add3/2  "D"
  Complex to Real-Imag1/1 -> D2_4/1, Add3/1  "C"
  In2/1 -> D1_2/1
  Real-Imag to Complex/1 -> Out1/1

== matlab function mvdr_4x4_partial_systolic/MVDR HDL/Compute Weight Vector/Serialize Input Data/readyQueue ==
  data: readyEdge input; validOut output; validIn input
function validOut = readyQueue(readyEdge, validIn)

persistent readyQueued_reg
if isempty(readyQueued_reg)
    readyQueued_reg = false;
end

readyQueued = readyQueued_reg;

if readyEdge
    if validIn
        validOut = true;
    else
        validOut = false;
        readyQueued_reg = true;
    end
elseif readyQueued
    if validIn
        validOut = true;
        readyQueued_reg = false;
    else
        validOut = false; 
    end
else
    validOut = false;
end

== matlab function mvdr_4x4_partial_systolic/MVDR HDL/Moving Average/Window Delay/Delay Enabled Synchronous RAM Based/Zero on Initial Delay/Zeros Like ==
  settings: fimath=hdlfimath
  data: u input; y output; matchInputSize parameter; outputSize parameter
function y = zeros_like(u, matchInputSize, outputSize)

if matchInputSize
    y = zeros(size(u),'like',u);
else
    y = zeros(outputSize,'like',u);
end

== matlab function mvdr_4x4_partial_systolic/MVDR HDL/Diagonal Loading/Generate Loading Eye Matrix ==
  data: in input; out output; numArrayElements parameter
function out = gen_eye(in,numArrayElements)

temp = zeros([numArrayElements numArrayElements],'like',in);
coder.unroll();
for ii=1:numArrayElements
    temp(ii,ii) = in;
end

out = temp;
